simulink model "Motor"  (R2025a)
settings: Solver=VariableStepAuto  StartTime=0.0  StopTime=10.0  RelTol=1e-3
undefined symbols (not defined in the file): Im, Km, Kw, Ra, Te
settings Model: Creator=Имя  LastModifiedBy=Имя

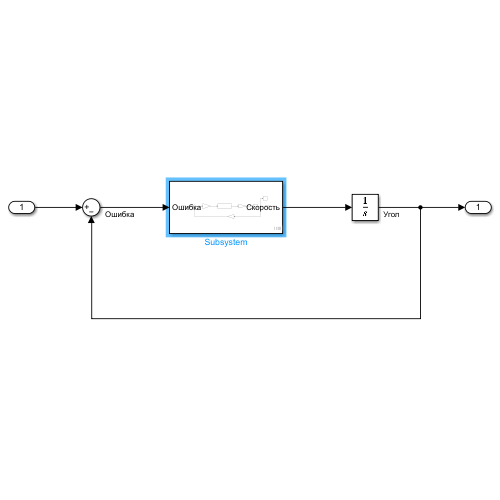
[thumbnail: Simulink's stored preview of the top-level diagram]
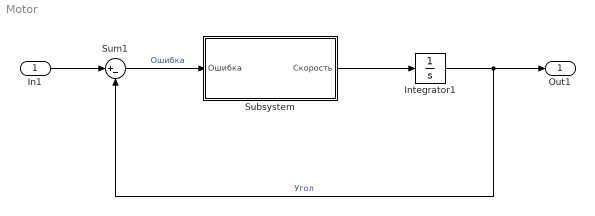
== system Motor ==
  In1 : Inport
  Integrator1 : Integrator
  Subsystem : Subsystem
  Sum1 : Sum  Inputs=|+-
  Out1 : Outport
  wires:
  Integrator1/1 -> Out1/1, Sum1/2  "Угол"
  In1/1 -> Sum1/1
  Sum1/1 -> Subsystem/1(Ошибка)  "Ошибка"
  Subsystem/1(Скорость) -> Integrator1/1

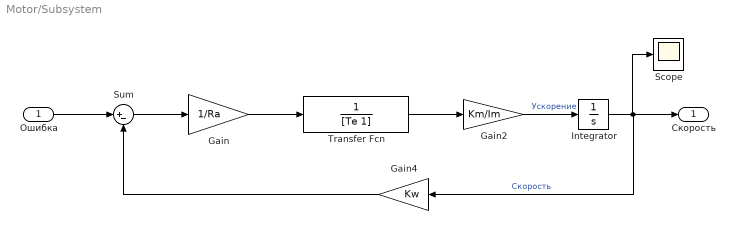
== system Motor/Subsystem ==
  Ошибка : Inport
  Gain : Gain  Gain=1/Ra
  Gain2 : Gain  Gain=Km/Im
  Gain4 : Gain  Gain=Kw
  Integrator : Integrator
  Scope : Scope
  Sum : Sum  Inputs=|+-
  Transfer Fcn : TransferFcn  Denominator=[Te 1]
  Скорость : Outport
  wires:
  Ошибка/1 -> Sum/1
  Sum/1 -> Gain/1
  Gain2/1 -> Integrator/1  "Ускорение"
  Transfer Fcn/1 -> Gain2/1
  Integrator/1 -> Scope/1, Скорость/1, Gain4/1  "Скорость"
  Gain/1 -> Transfer Fcn/1
  Gain4/1 -> Sum/2
